simulink model "Ejercicio31"  (R2023b)
settings: Solver=VariableStepAuto  StartTime=0.0  StopTime=8  RelTol=1e-3
settings Model: Creator=mende  LastModifiedBy=mende

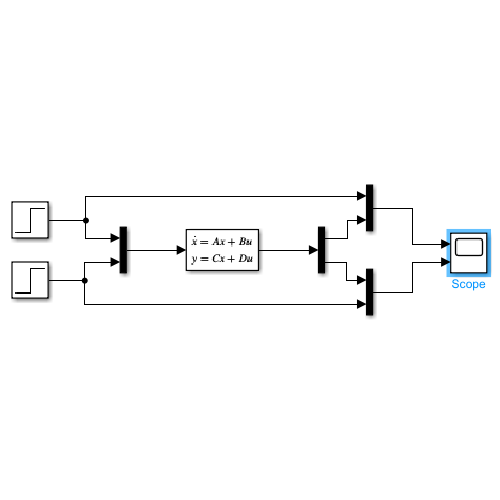
[thumbnail: Simulink's stored preview of the top-level diagram]
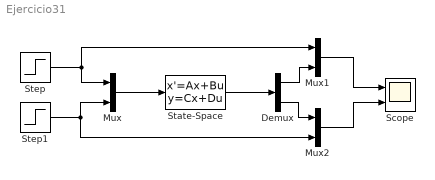
== system Ejercicio31 ==
  Demux : Demux  Outputs=2
  Mux : Mux  Inputs=2
  Mux1 : Mux  Inputs=2
  Mux2 : Mux  Inputs=2
  Scope : Scope  NumInputPorts=2
  State-Space : StateSpace  A=[0 1;-25 -4]  B=[1 1; 0 1]  C=[1 0; 0 1]  D=[0 0; 0 0]  InitialCondition=0  ParameterTunability=Optimized
  Step : Step  SampleTime=0
  Step1 : Step  SampleTime=0
  wires:
  Step/1 -> Mux/1, Mux1/1
  Mux/1 -> State-Space/1
  State-Space/1 -> Demux/1
  Demux/2 -> Mux2/1
  Demux/1 -> Mux1/2
  Step1/1 -> Mux2/2, Mux/2
  Mux1/1 -> Scope/1
  Mux2/1 -> Scope/2
